simulink model "dft_8_point"  (R2016b)
settings: Solver=VariableStepDiscrete  StartTime=0.0  StopTime=12/fs  RelTol=1e-3  EnableMultiTasking=on
PreLoadFcn:
  | t = 2;
  | b = 14;
  | 
  | fs = 1;
StartFcn:
  | close all;
StopFcn:
  | % create matrices of Re and Im parts over time - inputs
  | xin_re = [xin_0_re xin_1_re xin_2_re xin_3_re xin_4_re xin_5_re xin_6_re xin_7_re];
  | xin_im = [xin_0_im xin_0_im xin_0_im xin_0_im xin_0_im xin_0_im xin_0_im xin_0_im];
  | 
  | % create matrices of Re and Im parts over time - outputs
  | X_re = [X0_re X1_re X2_re X3_re X4_re X5_re X6_re X7_re];
  | X_im = [X0_im X1_im X2_im X3_im X4_im X5_im X6_im X7_im];
  | 
  | % create vectors of Magnitudes and Angles over time
  | X_mag = [X0_mag X1_mag X2_mag X3_mag X4_mag X5_mag X6_mag X7_mag];
  | X_ang = [X0_ang X1_ang X2_ang X3_ang X4_ang X5_ang X6_ang X7_ang];
  | 
  | 
  | figure(1)
  | hold off
  | plot([0:1:7],xin_re(end,:),'r-o','MarkerFaceColor','r');
  | hold on
  | plot([0:1:7],xin_im(end,:),'b-o','MarkerFaceColor','b');
  | xlabel('Samples');
  | ylabel('Magnitude');
  | title('Input to DFT');
  | legend('Real','Imaginary','Location','EastOutside')
  | grid on;
  | 
  | set(1,'Name','Input to DFT','NumberTitle','off');
  | % setStandardFigSize(1);
  | 
  | figure(2)
  | hold off
  | plot([0:1:7],X_mag(end,:),'k-o','MarkerFaceColor','b');
  | hold on
  | xlabel('Frequency Bin');
  | ylabel('Magnitude');
  | grid on;
  | title('Magnitude DFT Plot');
  | 
  | set(2,'Name','Output of DFT','NumberTitle','off');
  | % setStandardFigSize(2);
libraries: xbsIndex_r4 x955
(part 2 of 8)

== system dft_8_point/Capture X0 Outputs ==
  In1 : Inport
  In2 : Inport  Port=2
  Complex to Magnitude-Angle : ComplexToMagnitudeAngle
  Real-Imag to Complex : RealImagToComplex
  To Workspace : ToWorkspace  VariableName=X0_im  SampleTime=-1
  To Workspace1 : ToWorkspace  VariableName=X0_re  SampleTime=-1
  To Workspace16 : ToWorkspace  VariableName=X0_mag  SampleTime=-1
  To Workspace17 : ToWorkspace  VariableName=X0_ang  SampleTime=-1
  wires:
  In1/1 -> Real-Imag to Complex/2, To Workspace/1
  In2/1 -> Real-Imag to Complex/1, To Workspace1/1
  Real-Imag to Complex/1 -> Complex to Magnitude-Angle/1
  Complex to Magnitude-Angle/2 -> To Workspace17/1
  Complex to Magnitude-Angle/1 -> To Workspace16/1

== system dft_8_point/Capture X2 Outputs ==
  In1 : Inport
  In2 : Inport  Port=2
  Complex to Magnitude-Angle2 : ComplexToMagnitudeAngle
  Real-Imag to Complex2 : RealImagToComplex
  To Workspace20 : ToWorkspace  VariableName=X2_mag  SampleTime=-1
  To Workspace21 : ToWorkspace  VariableName=X2_ang  SampleTime=-1
  To Workspace4 : ToWorkspace  VariableName=X2_im  SampleTime=-1
  To Workspace5 : ToWorkspace  VariableName=X2_re  SampleTime=-1
  wires:
  In1/1 -> Real-Imag to Complex2/2, To Workspace4/1
  In2/1 -> Real-Imag to Complex2/1, To Workspace5/1
  Real-Imag to Complex2/1 -> Complex to Magnitude-Angle2/1
  Complex to Magnitude-Angle2/2 -> To Workspace21/1
  Complex to Magnitude-Angle2/1 -> To Workspace20/1

== system dft_8_point/Capture X6 Outputs ==
  In1 : Inport
  In2 : Inport  Port=2
  Complex to Magnitude-Angle6 : ComplexToMagnitudeAngle
  Real-Imag to Complex6 : RealImagToComplex
  To Workspace12 : ToWorkspace  VariableName=X6_im  SampleTime=-1
  To Workspace13 : ToWorkspace  VariableName=X6_re  SampleTime=-1
  To Workspace28 : ToWorkspace  VariableName=X6_mag  SampleTime=-1
  To Workspace29 : ToWorkspace  VariableName=X6_ang  SampleTime=-1
  wires:
  In1/1 -> Real-Imag to Complex6/2, To Workspace12/1
  In2/1 -> Real-Imag to Complex6/1, To Workspace13/1
  Real-Imag to Complex6/1 -> Complex to Magnitude-Angle6/1
  Complex to Magnitude-Angle6/2 -> To Workspace29/1
  Complex to Magnitude-Angle6/1 -> To Workspace28/1

== system dft_8_point/Capture X1 Outputs ==
  In1 : Inport
  In2 : Inport  Port=2
  Complex to Magnitude-Angle1 : ComplexToMagnitudeAngle
  Real-Imag to Complex1 : RealImagToComplex
  To Workspace18 : ToWorkspace  VariableName=X1_mag  SampleTime=-1
  To Workspace19 : ToWorkspace  VariableName=X1_ang  SampleTime=-1
  To Workspace2 : ToWorkspace  VariableName=X1_im  SampleTime=-1
  To Workspace3 : ToWorkspace  VariableName=X1_re  SampleTime=-1
  wires:
  In1/1 -> Real-Imag to Complex1/2, To Workspace2/1
  In2/1 -> Real-Imag to Complex1/1, To Workspace3/1
  Real-Imag to Complex1/1 -> Complex to Magnitude-Angle1/1
  Complex to Magnitude-Angle1/2 -> To Workspace19/1
  Complex to Magnitude-Angle1/1 -> To Workspace18/1

== system dft_8_point/Capture X3 Outputs ==
  In1 : Inport
  In2 : Inport  Port=2
  Complex to Magnitude-Angle3 : ComplexToMagnitudeAngle
  Real-Imag to Complex3 : RealImagToComplex
  To Workspace22 : ToWorkspace  VariableName=X3_mag  SampleTime=-1
  To Workspace23 : ToWorkspace  VariableName=X3_ang  SampleTime=-1
  To Workspace6 : ToWorkspace  VariableName=X3_im  SampleTime=-1
  To Workspace7 : ToWorkspace  VariableName=X3_re  SampleTime=-1
  wires:
  In1/1 -> Real-Imag to Complex3/2, To Workspace6/1
  In2/1 -> Real-Imag to Complex3/1, To Workspace7/1
  Real-Imag to Complex3/1 -> Complex to Magnitude-Angle3/1
  Complex to Magnitude-Angle3/2 -> To Workspace23/1
  Complex to Magnitude-Angle3/1 -> To Workspace22/1

== system dft_8_point/Capture X4 Outputs ==
  In1 : Inport
  In2 : Inport  Port=2
  Complex to Magnitude-Angle4 : ComplexToMagnitudeAngle
  Real-Imag to Complex4 : RealImagToComplex
  To Workspace24 : ToWorkspace  VariableName=X4_mag  SampleTime=-1
  To Workspace25 : ToWorkspace  VariableName=X4_ang  SampleTime=-1
  To Workspace8 : ToWorkspace  VariableName=X4_im  SampleTime=-1
  To Workspace9 : ToWorkspace  VariableName=X4_re  SampleTime=-1
  wires:
  In1/1 -> Real-Imag to Complex4/2, To Workspace8/1
  In2/1 -> Real-Imag to Complex4/1, To Workspace9/1
  Real-Imag to Complex4/1 -> Complex to Magnitude-Angle4/1
  Complex to Magnitude-Angle4/2 -> To Workspace25/1
  Complex to Magnitude-Angle4/1 -> To Workspace24/1

== system dft_8_point/Capture X5 Outputs ==
  In1 : Inport
  In2 : Inport  Port=2
  Complex to Magnitude-Angle5 : ComplexToMagnitudeAngle
  Real-Imag to Complex5 : RealImagToComplex
  To Workspace10 : ToWorkspace  VariableName=X5_im  SampleTime=-1
  To Workspace11 : ToWorkspace  VariableName=X5_re  SampleTime=-1
  To Workspace26 : ToWorkspace  VariableName=X5_mag  SampleTime=-1
  To Workspace27 : ToWorkspace  VariableName=X5_ang  SampleTime=-1
  wires:
  In1/1 -> Real-Imag to Complex5/2, To Workspace10/1
  In2/1 -> Real-Imag to Complex5/1, To Workspace11/1
  Real-Imag to Complex5/1 -> Complex to Magnitude-Angle5/1
  Complex to Magnitude-Angle5/2 -> To Workspace27/1
  Complex to Magnitude-Angle5/1 -> To Workspace26/1

== system dft_8_point/Capture X7 Outputs ==
  In1 : Inport
  In2 : Inport  Port=2
  Complex to Magnitude-Angle7 : ComplexToMagnitudeAngle
  Real-Imag to Complex7 : RealImagToComplex
  To Workspace14 : ToWorkspace  VariableName=X7_im  SampleTime=-1
  To Workspace15 : ToWorkspace  VariableName=X7_re  SampleTime=-1
  To Workspace30 : ToWorkspace  VariableName=X7_mag  SampleTime=-1
  To Workspace31 : ToWorkspace  VariableName=X7_ang  SampleTime=-1
  wires:
  In1/1 -> Real-Imag to Complex7/2, To Workspace14/1
  In2/1 -> Real-Imag to Complex7/1, To Workspace15/1
  Real-Imag to Complex7/1 -> Complex to Magnitude-Angle7/1
  Complex to Magnitude-Angle7/2 -> To Workspace31/1
  Complex to Magnitude-Angle7/1 -> To Workspace30/1

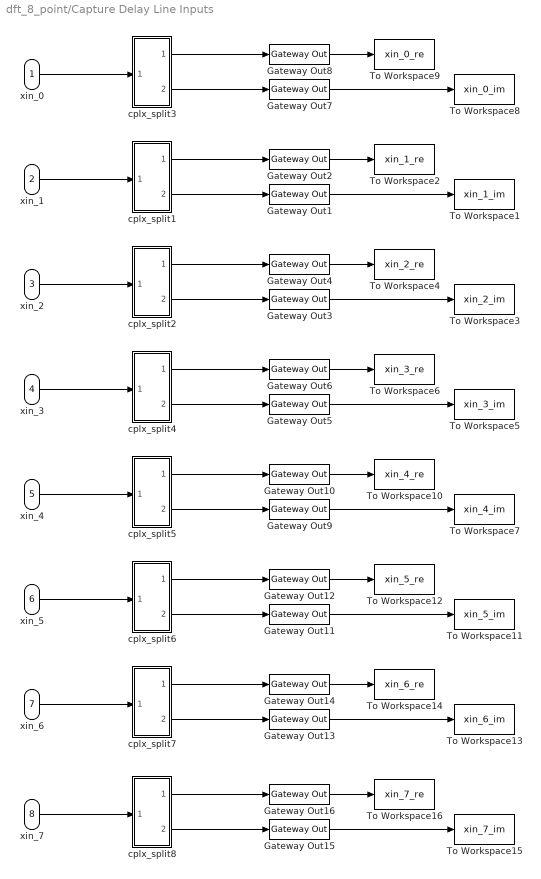
== system dft_8_point/Capture Delay Line Inputs ==
  xin_0 : Inport
  xin_1 : Inport  Port=2
  xin_2 : Inport  Port=3
  xin_3 : Inport  Port=4
  xin_4 : Inport  Port=5
  xin_5 : Inport  Port=6
  xin_6 : Inport  Port=7
  xin_7 : Inport  Port=8
  Gateway Out{1..16} (16 alike) : xbsIndex_r4/Gateway Out  inherit_from_input=off  hdl_port=off  rows=1  columns=1  UseAsDAC=off  DACChannel='1'  interface=None  automatic_assignment=on  address_offset=hex2dec('00')  intf_name=''  intf_description=''  timing_constraint=None  locs_specified=off  LOCs={}  io_standard={}  block_type=gatewayout
      settings: infoedit="Gateway out block.  Converts Xilinx fixed point inputs into ouputs of type Simulink integer, double, or fixed point.<br><br>Hardware notes:  In hardware these blocks become top level output ports or are discarded, depending on how they are configured."
  To Workspace1 : ToWorkspace  VariableName=xin_1_im  SampleTime=-1
  To Workspace10 : ToWorkspace  VariableName=xin_4_re  SampleTime=-1
  To Workspace11 : ToWorkspace  VariableName=xin_5_im  SampleTime=-1
  To Workspace12 : ToWorkspace  VariableName=xin_5_re  SampleTime=-1
  To Workspace13 : ToWorkspace  VariableName=xin_6_im  SampleTime=-1
  To Workspace14 : ToWorkspace  VariableName=xin_6_re  SampleTime=-1
  To Workspace15 : ToWorkspace  VariableName=xin_7_im  SampleTime=-1
  To Workspace16 : ToWorkspace  VariableName=xin_7_re  SampleTime=-1
  To Workspace2 : ToWorkspace  VariableName=xin_1_re  SampleTime=-1
  To Workspace3 : ToWorkspace  VariableName=xin_2_im  SampleTime=-1
  To Workspace4 : ToWorkspace  VariableName=xin_2_re  SampleTime=-1
  To Workspace5 : ToWorkspace  VariableName=xin_3_im  SampleTime=-1
  To Workspace6 : ToWorkspace  VariableName=xin_3_re  SampleTime=-1
  To Workspace7 : ToWorkspace  VariableName=xin_4_im  SampleTime=-1
  To Workspace8 : ToWorkspace  VariableName=xin_0_im  SampleTime=-1
  To Workspace9 : ToWorkspace  VariableName=xin_0_re  SampleTime=-1
  cplx_split1 : Subsystem  mask(Complex to Real / Imaginary){t=t, b=b}
      mask prompts: t "Input integer bits"; b "Input fractional bits"
      mask help:
      | This block converts the signal from a signal complex one {real,imaginary} to separate parts.
      |
      | The integer and fractional wordlengths of the real and imaginary parts are supplied so that the combined word can be separated.
  cplx_split2 : Subsystem  mask(Complex to Real / Imaginary){t=t, b=b}
      mask prompts: t "Input integer bits"; b "Input fractional bits"
      mask help:
      | This block converts the signal from a signal complex one {real,imaginary} to separate parts.
      |
      | The integer and fractional wordlengths of the real and imaginary parts are supplied so that the combined word can be separated.
  cplx_split3 : Subsystem  mask(Complex to Real / Imaginary){t=t, b=b}
      mask prompts: t "Input integer bits"; b "Input fractional bits"
      mask help:
      | This block converts the signal from a signal complex one {real,imaginary} to separate parts.
      |
      | The integer and fractional wordlengths of the real and imaginary parts are supplied so that the combined word can be separated.
  cplx_split4 : Subsystem  mask(Complex to Real / Imaginary){t=t, b=b}
      mask prompts: t "Input integer bits"; b "Input fractional bits"
      mask help:
      | This block converts the signal from a signal complex one {real,imaginary} to separate parts.
      |
      | The integer and fractional wordlengths of the real and imaginary parts are supplied so that the combined word can be separated.
  cplx_split5 : Subsystem  mask(Complex to Real / Imaginary){t=t, b=b}
      mask prompts: t "Input integer bits"; b "Input fractional bits"
      mask help:
      | This block converts the signal from a signal complex one {real,imaginary} to separate parts.
      |
      | The integer and fractional wordlengths of the real and imaginary parts are supplied so that the combined word can be separated.
  cplx_split6 : Subsystem  mask(Complex to Real / Imaginary){t=t, b=b}
      mask prompts: t "Input integer bits"; b "Input fractional bits"
      mask help:
      | This block converts the signal from a signal complex one {real,imaginary} to separate parts.
      |
      | The integer and fractional wordlengths of the real and imaginary parts are supplied so that the combined word can be separated.
  cplx_split7 : Subsystem  mask(Complex to Real / Imaginary){t=t, b=b}
      mask prompts: t "Input integer bits"; b "Input fractional bits"
      mask help:
      | This block converts the signal from a signal complex one {real,imaginary} to separate parts.
      |
      | The integer and fractional wordlengths of the real and imaginary parts are supplied so that the combined word can be separated.
  cplx_split8 : Subsystem  mask(Complex to Real / Imaginary){t=t, b=b}
      mask prompts: t "Input integer bits"; b "Input fractional bits"
      mask help:
      | This block converts the signal from a signal complex one {real,imaginary} to separate parts.
      |
      | The integer and fractional wordlengths of the real and imaginary parts are supplied so that the combined word can be separated.
  wires:
  xin_0/1 -> cplx_split3/1(cmplx)
  xin_1/1 -> cplx_split1/1(cmplx)
  xin_2/1 -> cplx_split2/1(cmplx)
  xin_3/1 -> cplx_split4/1(cmplx)
  xin_4/1 -> cplx_split5/1(cmplx)
  xin_5/1 -> cplx_split6/1(cmplx)
  xin_6/1 -> cplx_split7/1(cmplx)
  xin_7/1 -> cplx_split8/1(cmplx)
  cplx_split3/1(real) -> Gateway Out8/1
  cplx_split3/2(imag) -> Gateway Out7/1
  Gateway Out7/1 -> To Workspace8/1
  Gateway Out8/1 -> To Workspace9/1
  cplx_split1/1(real) -> Gateway Out2/1
  cplx_split1/2(imag) -> Gateway Out1/1
  Gateway Out1/1 -> To Workspace1/1
  Gateway Out2/1 -> To Workspace2/1
  cplx_split2/1(real) -> Gateway Out4/1
  cplx_split2/2(imag) -> Gateway Out3/1
  Gateway Out3/1 -> To Workspace3/1
  Gateway Out4/1 -> To Workspace4/1
  cplx_split4/1(real) -> Gateway Out6/1
  cplx_split4/2(imag) -> Gateway Out5/1
  Gateway Out5/1 -> To Workspace5/1
  Gateway Out6/1 -> To Workspace6/1
  cplx_split5/1(real) -> Gateway Out10/1
  cplx_split5/2(imag) -> Gateway Out9/1
  Gateway Out9/1 -> To Workspace7/1
  Gateway Out10/1 -> To Workspace10/1
  cplx_split6/1(real) -> Gateway Out12/1
  cplx_split6/2(imag) -> Gateway Out11/1
  Gateway Out11/1 -> To Workspace11/1
  Gateway Out12/1 -> To Workspace12/1
  cplx_split7/1(real) -> Gateway Out14/1
  cplx_split7/2(imag) -> Gateway Out13/1
  Gateway Out13/1 -> To Workspace13/1
  Gateway Out14/1 -> To Workspace14/1
  cplx_split8/1(real) -> Gateway Out16/1
  cplx_split8/2(imag) -> Gateway Out15/1
  Gateway Out15/1 -> To Workspace15/1
  Gateway Out16/1 -> To Workspace16/1

== system dft_8_point/See: File -> Model Properties -> Callbacks -> PreLoadFcn  ==

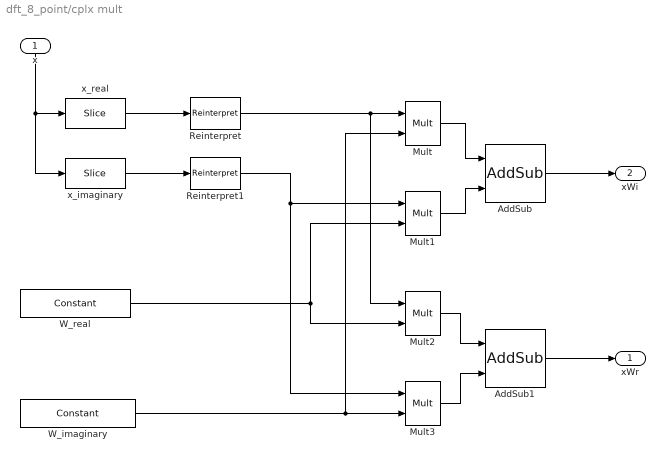
== system dft_8_point/cplx mult ==
  x : Inport
  AddSub : xbsIndex_r4/AddSub  mode=Addition  use_carryin=off  use_carryout=off  en=off  latency=0  precision=User Defined  arith_type="Signed  (2's comp)"  n_bits=t+b+1  bin_pt=b  quantization=Truncate  overflow=Wrap  use_behavioral_HDL=off  hw_selection=Fabric  pipelined=off  dbl_ovrd=off  block_type=addsub
  AddSub1 : xbsIndex_r4/AddSub  mode=Subtraction  use_carryin=off  use_carryout=off  en=off  latency=0  precision=User Defined  arith_type="Signed  (2's comp)"  n_bits=t+b+1  bin_pt=b  quantization=Truncate  overflow=Wrap  use_behavioral_HDL=off  hw_selection=Fabric  pipelined=off  dbl_ovrd=off  block_type=addsub
  Mult{,1..3} (4 alike) : xbsIndex_r4/Mult  precision=User Defined  arith_type="Signed  (2's comp)"  n_bits=t+b  bin_pt=b  quantization=Truncate  overflow=Wrap  en=off  latency=0  use_behavioral_HDL=off  opt=Speed  use_embedded=on  optimum_pipeline=off  pipeline=on  dbl_ovrd=off  use_rpm=on  placement_style=Triangular  block_type=mult
  Reinterpret : xbsIndex_r4/Reinterpret  force_arith_type=on  arith_type="Signed  (2's comp)"  force_bin_pt=on  bin_pt=b  block_type=reinterpret
      settings: infoedit="Changes signal type without altering the binary representation.   You can changed the signal between signed and unsigned, and relocate the binary point.<br><br>Hardware notes: In hardware this block costs nothing.<br><br>Example:  Suppose the input is 6 bits wide, signed, with 2 fractional bits, and the output is forced to unsigned with 0 fractional bits.  Then an input of -2.0 (1110.00 in binary 2's complement) becomes an output of 56 (111000 in binary)."
  Reinterpret1 : xbsIndex_r4/Reinterpret  force_arith_type=on  arith_type="Signed  (2's comp)"  force_bin_pt=on  bin_pt=b  block_type=reinterpret
      settings: infoedit="Changes signal type without altering the binary representation.   You can changed the signal between signed and unsigned, and relocate the binary point.<br><br>Hardware notes: In hardware this block costs nothing.<br><br>Example:  Suppose the input is 6 bits wide, signed, with 2 fractional bits, and the output is forced to unsigned with 0 fractional bits.  Then an input of -2.0 (1110.00 in binary 2's complement) becomes an output of 56 (111000 in binary)."
  W_imaginary : xbsIndex_r4/Constant  const=imag(Wnk)  gui_display_data_type=Fixed-point  arith_type=Signed (2's comp)  n_bits=t+b  bin_pt=b  preci_type=Single  exp_width=8  frac_width=24  explicit_period=off  period=1  equ=P=C  opselect=C  inp2=PCIN>>17  opr=+  inp1=P  carry=CIN  dbl_ovrd=off  block_type=constant
  W_real : xbsIndex_r4/Constant  const=real(Wnk)  gui_display_data_type=Fixed-point  arith_type=Signed (2's comp)  n_bits=t+b  bin_pt=b  preci_type=Single  exp_width=8  frac_width=24  explicit_period=off  period=1  equ=P=C  opselect=C  inp2=PCIN>>17  opr=+  inp1=P  carry=CIN  dbl_ovrd=off  block_type=constant
  x_imaginary : xbsIndex_r4/Slice  nbits=t+b  boolean_output=off  mode=Lower Bit Location + Width  bit1=0  base1=MSB of Input  bit0=0  base0=LSB of Input  dbl_ovrd=off  block_type=slice
  x_real : xbsIndex_r4/Slice  nbits=t+b  boolean_output=off  mode=Upper Bit Location + Width  bit1=0  base1=MSB of Input  bit0=0  base0=LSB of Input  dbl_ovrd=off  block_type=slice
  xWr : Outport
  xWi : Outport  Port=2
  wires:
  x_real/1 -> Reinterpret/1
  x_imaginary/1 -> Reinterpret1/1
  W_real/1 -> Mult1/2, Mult2/2
  x/1 -> x_real/1, x_imaginary/1
  Reinterpret/1 -> Mult/1, Mult2/1
  Reinterpret1/1 -> Mult1/1, Mult3/1
  W_imaginary/1 -> Mult/2, Mult3/2
  AddSub/1 -> xWi/1
  AddSub1/1 -> xWr/1
  Mult/1 -> AddSub/1
  Mult1/1 -> AddSub/2
  Mult3/1 -> AddSub1/2
  Mult2/1 -> AddSub1/1

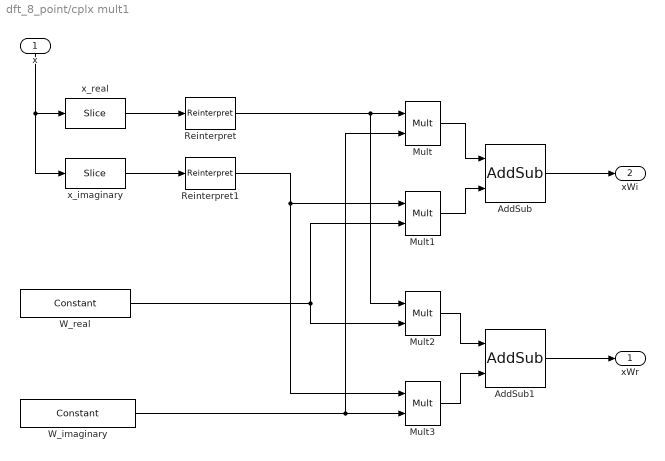
== system dft_8_point/cplx mult1 ==
  x : Inport
  AddSub : xbsIndex_r4/AddSub  mode=Addition  use_carryin=off  use_carryout=off  en=off  latency=0  precision=User Defined  arith_type="Signed  (2's comp)"  n_bits=t+b+1  bin_pt=b  quantization=Truncate  overflow=Wrap  use_behavioral_HDL=off  hw_selection=Fabric  pipelined=off  dbl_ovrd=off  block_type=addsub
  AddSub1 : xbsIndex_r4/AddSub  mode=Subtraction  use_carryin=off  use_carryout=off  en=off  latency=0  precision=User Defined  arith_type="Signed  (2's comp)"  n_bits=t+b+1  bin_pt=b  quantization=Truncate  overflow=Wrap  use_behavioral_HDL=off  hw_selection=Fabric  pipelined=off  dbl_ovrd=off  block_type=addsub
  Mult{,1..3} (4 alike) : xbsIndex_r4/Mult  precision=User Defined  arith_type="Signed  (2's comp)"  n_bits=t+b  bin_pt=b  quantization=Truncate  overflow=Wrap  en=off  latency=0  use_behavioral_HDL=off  opt=Speed  use_embedded=on  optimum_pipeline=off  pipeline=on  dbl_ovrd=off  use_rpm=on  placement_style=Triangular  block_type=mult
  Reinterpret : xbsIndex_r4/Reinterpret  force_arith_type=on  arith_type="Signed  (2's comp)"  force_bin_pt=on  bin_pt=b  block_type=reinterpret
      settings: infoedit="Changes signal type without altering the binary representation.   You can changed the signal between signed and unsigned, and relocate the binary point.<br><br>Hardware notes: In hardware this block costs nothing.<br><br>Example:  Suppose the input is 6 bits wide, signed, with 2 fractional bits, and the output is forced to unsigned with 0 fractional bits.  Then an input of -2.0 (1110.00 in binary 2's complement) becomes an output of 56 (111000 in binary)."
  Reinterpret1 : xbsIndex_r4/Reinterpret  force_arith_type=on  arith_type="Signed  (2's comp)"  force_bin_pt=on  bin_pt=b  block_type=reinterpret
      settings: infoedit="Changes signal type without altering the binary representation.   You can changed the signal between signed and unsigned, and relocate the binary point.<br><br>Hardware notes: In hardware this block costs nothing.<br><br>Example:  Suppose the input is 6 bits wide, signed, with 2 fractional bits, and the output is forced to unsigned with 0 fractional bits.  Then an input of -2.0 (1110.00 in binary 2's complement) becomes an output of 56 (111000 in binary)."
  W_imaginary : xbsIndex_r4/Constant  const=imag(Wnk)  gui_display_data_type=Fixed-point  arith_type=Signed (2's comp)  n_bits=t+b  bin_pt=b  preci_type=Single  exp_width=8  frac_width=24  explicit_period=off  period=1  equ=P=C  opselect=C  inp2=PCIN>>17  opr=+  inp1=P  carry=CIN  dbl_ovrd=off  block_type=constant
  W_real : xbsIndex_r4/Constant  const=real(Wnk)  gui_display_data_type=Fixed-point  arith_type=Signed (2's comp)  n_bits=t+b  bin_pt=b  preci_type=Single  exp_width=8  frac_width=24  explicit_period=off  period=1  equ=P=C  opselect=C  inp2=PCIN>>17  opr=+  inp1=P  carry=CIN  dbl_ovrd=off  block_type=constant
  x_imaginary : xbsIndex_r4/Slice  nbits=t+b  boolean_output=off  mode=Lower Bit Location + Width  bit1=0  base1=MSB of Input  bit0=0  base0=LSB of Input  dbl_ovrd=off  block_type=slice
  x_real : xbsIndex_r4/Slice  nbits=t+b  boolean_output=off  mode=Upper Bit Location + Width  bit1=0  base1=MSB of Input  bit0=0  base0=LSB of Input  dbl_ovrd=off  block_type=slice
  xWr : Outport
  xWi : Outport  Port=2
  wires:
  x_real/1 -> Reinterpret/1
  x_imaginary/1 -> Reinterpret1/1
  W_real/1 -> Mult1/2, Mult2/2
  x/1 -> x_real/1, x_imaginary/1
  Reinterpret/1 -> Mult/1, Mult2/1
  Reinterpret1/1 -> Mult1/1, Mult3/1
  W_imaginary/1 -> Mult/2, Mult3/2
  AddSub/1 -> xWi/1
  AddSub1/1 -> xWr/1
  Mult/1 -> AddSub/1
  Mult1/1 -> AddSub/2
  Mult3/1 -> AddSub1/2
  Mult2/1 -> AddSub1/1

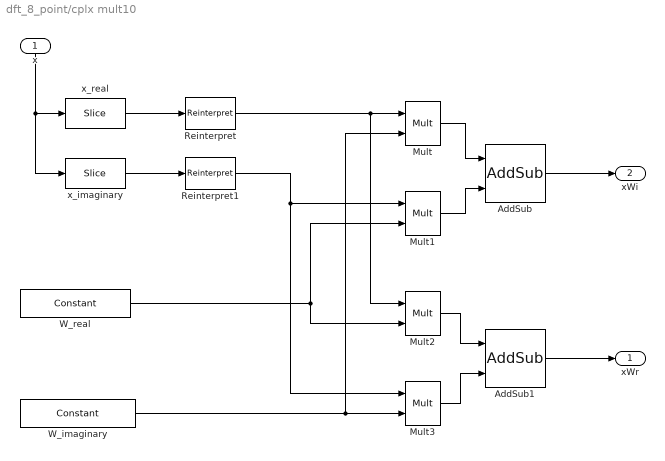
== system dft_8_point/cplx mult10 ==
  x : Inport
  AddSub : xbsIndex_r4/AddSub  mode=Addition  use_carryin=off  use_carryout=off  en=off  latency=0  precision=User Defined  arith_type="Signed  (2's comp)"  n_bits=t+b+1  bin_pt=b  quantization=Truncate  overflow=Wrap  use_behavioral_HDL=off  hw_selection=Fabric  pipelined=off  dbl_ovrd=off  block_type=addsub
  AddSub1 : xbsIndex_r4/AddSub  mode=Subtraction  use_carryin=off  use_carryout=off  en=off  latency=0  precision=User Defined  arith_type="Signed  (2's comp)"  n_bits=t+b+1  bin_pt=b  quantization=Truncate  overflow=Wrap  use_behavioral_HDL=off  hw_selection=Fabric  pipelined=off  dbl_ovrd=off  block_type=addsub
  Mult{,1..3} (4 alike) : xbsIndex_r4/Mult  precision=User Defined  arith_type="Signed  (2's comp)"  n_bits=t+b  bin_pt=b  quantization=Truncate  overflow=Wrap  en=off  latency=0  use_behavioral_HDL=off  opt=Speed  use_embedded=on  optimum_pipeline=off  pipeline=on  dbl_ovrd=off  use_rpm=on  placement_style=Triangular  block_type=mult
  Reinterpret : xbsIndex_r4/Reinterpret  force_arith_type=on  arith_type="Signed  (2's comp)"  force_bin_pt=on  bin_pt=b  block_type=reinterpret
      settings: infoedit="Changes signal type without altering the binary representation.   You can changed the signal between signed and unsigned, and relocate the binary point.<br><br>Hardware notes: In hardware this block costs nothing.<br><br>Example:  Suppose the input is 6 bits wide, signed, with 2 fractional bits, and the output is forced to unsigned with 0 fractional bits.  Then an input of -2.0 (1110.00 in binary 2's complement) becomes an output of 56 (111000 in binary)."
  Reinterpret1 : xbsIndex_r4/Reinterpret  force_arith_type=on  arith_type="Signed  (2's comp)"  force_bin_pt=on  bin_pt=b  block_type=reinterpret
      settings: infoedit="Changes signal type without altering the binary representation.   You can changed the signal between signed and unsigned, and relocate the binary point.<br><br>Hardware notes: In hardware this block costs nothing.<br><br>Example:  Suppose the input is 6 bits wide, signed, with 2 fractional bits, and the output is forced to unsigned with 0 fractional bits.  Then an input of -2.0 (1110.00 in binary 2's complement) becomes an output of 56 (111000 in binary)."
  W_imaginary : xbsIndex_r4/Constant  const=imag(Wnk)  gui_display_data_type=Fixed-point  arith_type=Signed (2's comp)  n_bits=t+b  bin_pt=b  preci_type=Single  exp_width=8  frac_width=24  explicit_period=off  period=1  equ=P=C  opselect=C  inp2=PCIN>>17  opr=+  inp1=P  carry=CIN  dbl_ovrd=off  block_type=constant
  W_real : xbsIndex_r4/Constant  const=real(Wnk)  gui_display_data_type=Fixed-point  arith_type=Signed (2's comp)  n_bits=t+b  bin_pt=b  preci_type=Single  exp_width=8  frac_width=24  explicit_period=off  period=1  equ=P=C  opselect=C  inp2=PCIN>>17  opr=+  inp1=P  carry=CIN  dbl_ovrd=off  block_type=constant
  x_imaginary : xbsIndex_r4/Slice  nbits=t+b  boolean_output=off  mode=Lower Bit Location + Width  bit1=0  base1=MSB of Input  bit0=0  base0=LSB of Input  dbl_ovrd=off  block_type=slice
  x_real : xbsIndex_r4/Slice  nbits=t+b  boolean_output=off  mode=Upper Bit Location + Width  bit1=0  base1=MSB of Input  bit0=0  base0=LSB of Input  dbl_ovrd=off  block_type=slice
  xWr : Outport
  xWi : Outport  Port=2
  wires:
  x_real/1 -> Reinterpret/1
  x_imaginary/1 -> Reinterpret1/1
  W_real/1 -> Mult1/2, Mult2/2
  x/1 -> x_real/1, x_imaginary/1
  Reinterpret/1 -> Mult/1, Mult2/1
  Reinterpret1/1 -> Mult1/1, Mult3/1
  W_imaginary/1 -> Mult/2, Mult3/2
  AddSub/1 -> xWi/1
  AddSub1/1 -> xWr/1
  Mult/1 -> AddSub/1
  Mult1/1 -> AddSub/2
  Mult3/1 -> AddSub1/2
  Mult2/1 -> AddSub1/1

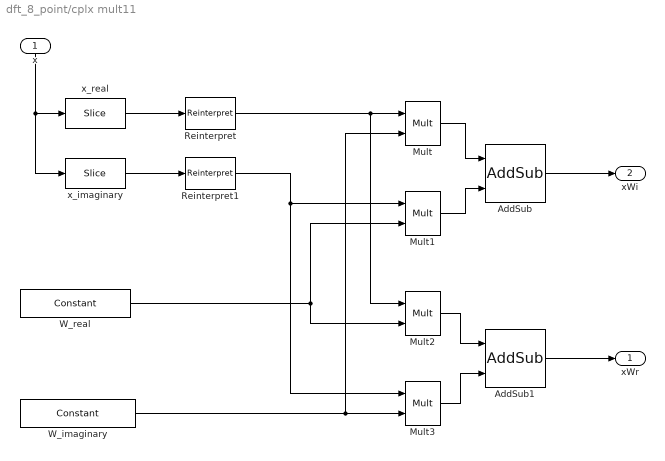
== system dft_8_point/cplx mult11 ==
  x : Inport
  AddSub : xbsIndex_r4/AddSub  mode=Addition  use_carryin=off  use_carryout=off  en=off  latency=0  precision=User Defined  arith_type="Signed  (2's comp)"  n_bits=t+b+1  bin_pt=b  quantization=Truncate  overflow=Wrap  use_behavioral_HDL=off  hw_selection=Fabric  pipelined=off  dbl_ovrd=off  block_type=addsub
  AddSub1 : xbsIndex_r4/AddSub  mode=Subtraction  use_carryin=off  use_carryout=off  en=off  latency=0  precision=User Defined  arith_type="Signed  (2's comp)"  n_bits=t+b+1  bin_pt=b  quantization=Truncate  overflow=Wrap  use_behavioral_HDL=off  hw_selection=Fabric  pipelined=off  dbl_ovrd=off  block_type=addsub
  Mult{,1..3} (4 alike) : xbsIndex_r4/Mult  precision=User Defined  arith_type="Signed  (2's comp)"  n_bits=t+b  bin_pt=b  quantization=Truncate  overflow=Wrap  en=off  latency=0  use_behavioral_HDL=off  opt=Speed  use_embedded=on  optimum_pipeline=off  pipeline=on  dbl_ovrd=off  use_rpm=on  placement_style=Triangular  block_type=mult
  Reinterpret : xbsIndex_r4/Reinterpret  force_arith_type=on  arith_type="Signed  (2's comp)"  force_bin_pt=on  bin_pt=b  block_type=reinterpret
      settings: infoedit="Changes signal type without altering the binary representation.   You can changed the signal between signed and unsigned, and relocate the binary point.<br><br>Hardware notes: In hardware this block costs nothing.<br><br>Example:  Suppose the input is 6 bits wide, signed, with 2 fractional bits, and the output is forced to unsigned with 0 fractional bits.  Then an input of -2.0 (1110.00 in binary 2's complement) becomes an output of 56 (111000 in binary)."
  Reinterpret1 : xbsIndex_r4/Reinterpret  force_arith_type=on  arith_type="Signed  (2's comp)"  force_bin_pt=on  bin_pt=b  block_type=reinterpret
      settings: infoedit="Changes signal type without altering the binary representation.   You can changed the signal between signed and unsigned, and relocate the binary point.<br><br>Hardware notes: In hardware this block costs nothing.<br><br>Example:  Suppose the input is 6 bits wide, signed, with 2 fractional bits, and the output is forced to unsigned with 0 fractional bits.  Then an input of -2.0 (1110.00 in binary 2's complement) becomes an output of 56 (111000 in binary)."
  W_imaginary : xbsIndex_r4/Constant  const=imag(Wnk)  gui_display_data_type=Fixed-point  arith_type=Signed (2's comp)  n_bits=t+b  bin_pt=b  preci_type=Single  exp_width=8  frac_width=24  explicit_period=off  period=1  equ=P=C  opselect=C  inp2=PCIN>>17  opr=+  inp1=P  carry=CIN  dbl_ovrd=off  block_type=constant
  W_real : xbsIndex_r4/Constant  const=real(Wnk)  gui_display_data_type=Fixed-point  arith_type=Signed (2's comp)  n_bits=t+b  bin_pt=b  preci_type=Single  exp_width=8  frac_width=24  explicit_period=off  period=1  equ=P=C  opselect=C  inp2=PCIN>>17  opr=+  inp1=P  carry=CIN  dbl_ovrd=off  block_type=constant
  x_imaginary : xbsIndex_r4/Slice  nbits=t+b  boolean_output=off  mode=Lower Bit Location + Width  bit1=0  base1=MSB of Input  bit0=0  base0=LSB of Input  dbl_ovrd=off  block_type=slice
  x_real : xbsIndex_r4/Slice  nbits=t+b  boolean_output=off  mode=Upper Bit Location + Width  bit1=0  base1=MSB of Input  bit0=0  base0=LSB of Input  dbl_ovrd=off  block_type=slice
  xWr : Outport
  xWi : Outport  Port=2
  wires:
  x_real/1 -> Reinterpret/1
  x_imaginary/1 -> Reinterpret1/1
  W_real/1 -> Mult1/2, Mult2/2
  x/1 -> x_real/1, x_imaginary/1
  Reinterpret/1 -> Mult/1, Mult2/1
  Reinterpret1/1 -> Mult1/1, Mult3/1
  W_imaginary/1 -> Mult/2, Mult3/2
  AddSub/1 -> xWi/1
  AddSub1/1 -> xWr/1
  Mult/1 -> AddSub/1
  Mult1/1 -> AddSub/2
  Mult3/1 -> AddSub1/2
  Mult2/1 -> AddSub1/1

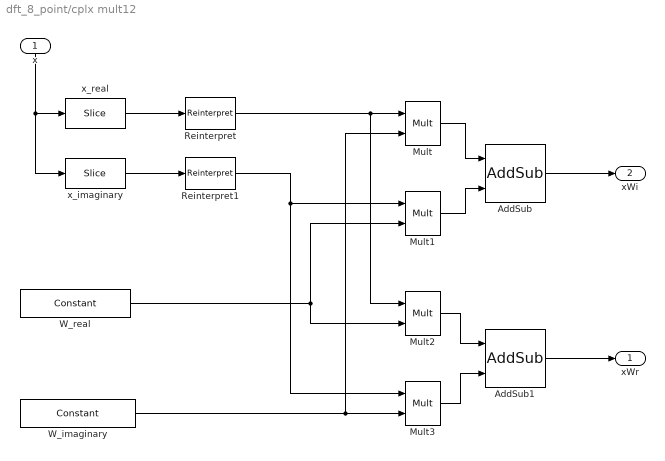
== system dft_8_point/cplx mult12 ==
  x : Inport
  AddSub : xbsIndex_r4/AddSub  mode=Addition  use_carryin=off  use_carryout=off  en=off  latency=0  precision=User Defined  arith_type="Signed  (2's comp)"  n_bits=t+b+1  bin_pt=b  quantization=Truncate  overflow=Wrap  use_behavioral_HDL=off  hw_selection=Fabric  pipelined=off  dbl_ovrd=off  block_type=addsub
  AddSub1 : xbsIndex_r4/AddSub  mode=Subtraction  use_carryin=off  use_carryout=off  en=off  latency=0  precision=User Defined  arith_type="Signed  (2's comp)"  n_bits=t+b+1  bin_pt=b  quantization=Truncate  overflow=Wrap  use_behavioral_HDL=off  hw_selection=Fabric  pipelined=off  dbl_ovrd=off  block_type=addsub
  Mult{,1..3} (4 alike) : xbsIndex_r4/Mult  precision=User Defined  arith_type="Signed  (2's comp)"  n_bits=t+b  bin_pt=b  quantization=Truncate  overflow=Wrap  en=off  latency=0  use_behavioral_HDL=off  opt=Speed  use_embedded=on  optimum_pipeline=off  pipeline=on  dbl_ovrd=off  use_rpm=on  placement_style=Triangular  block_type=mult
  Reinterpret : xbsIndex_r4/Reinterpret  force_arith_type=on  arith_type="Signed  (2's comp)"  force_bin_pt=on  bin_pt=b  block_type=reinterpret
      settings: infoedit="Changes signal type without altering the binary representation.   You can changed the signal between signed and unsigned, and relocate the binary point.<br><br>Hardware notes: In hardware this block costs nothing.<br><br>Example:  Suppose the input is 6 bits wide, signed, with 2 fractional bits, and the output is forced to unsigned with 0 fractional bits.  Then an input of -2.0 (1110.00 in binary 2's complement) becomes an output of 56 (111000 in binary)."
  Reinterpret1 : xbsIndex_r4/Reinterpret  force_arith_type=on  arith_type="Signed  (2's comp)"  force_bin_pt=on  bin_pt=b  block_type=reinterpret
      settings: infoedit="Changes signal type without altering the binary representation.   You can changed the signal between signed and unsigned, and relocate the binary point.<br><br>Hardware notes: In hardware this block costs nothing.<br><br>Example:  Suppose the input is 6 bits wide, signed, with 2 fractional bits, and the output is forced to unsigned with 0 fractional bits.  Then an input of -2.0 (1110.00 in binary 2's complement) becomes an output of 56 (111000 in binary)."
  W_imaginary : xbsIndex_r4/Constant  const=imag(Wnk)  gui_display_data_type=Fixed-point  arith_type=Signed (2's comp)  n_bits=t+b  bin_pt=b  preci_type=Single  exp_width=8  frac_width=24  explicit_period=off  period=1  equ=P=C  opselect=C  inp2=PCIN>>17  opr=+  inp1=P  carry=CIN  dbl_ovrd=off  block_type=constant
  W_real : xbsIndex_r4/Constant  const=real(Wnk)  gui_display_data_type=Fixed-point  arith_type=Signed (2's comp)  n_bits=t+b  bin_pt=b  preci_type=Single  exp_width=8  frac_width=24  explicit_period=off  period=1  equ=P=C  opselect=C  inp2=PCIN>>17  opr=+  inp1=P  carry=CIN  dbl_ovrd=off  block_type=constant
  x_imaginary : xbsIndex_r4/Slice  nbits=t+b  boolean_output=off  mode=Lower Bit Location + Width  bit1=0  base1=MSB of Input  bit0=0  base0=LSB of Input  dbl_ovrd=off  block_type=slice
  x_real : xbsIndex_r4/Slice  nbits=t+b  boolean_output=off  mode=Upper Bit Location + Width  bit1=0  base1=MSB of Input  bit0=0  base0=LSB of Input  dbl_ovrd=off  block_type=slice
  xWr : Outport
  xWi : Outport  Port=2
  wires:
  x_real/1 -> Reinterpret/1
  x_imaginary/1 -> Reinterpret1/1
  W_real/1 -> Mult1/2, Mult2/2
  x/1 -> x_real/1, x_imaginary/1
  Reinterpret/1 -> Mult/1, Mult2/1
  Reinterpret1/1 -> Mult1/1, Mult3/1
  W_imaginary/1 -> Mult/2, Mult3/2
  AddSub/1 -> xWi/1
  AddSub1/1 -> xWr/1
  Mult/1 -> AddSub/1
  Mult1/1 -> AddSub/2
  Mult3/1 -> AddSub1/2
  Mult2/1 -> AddSub1/1

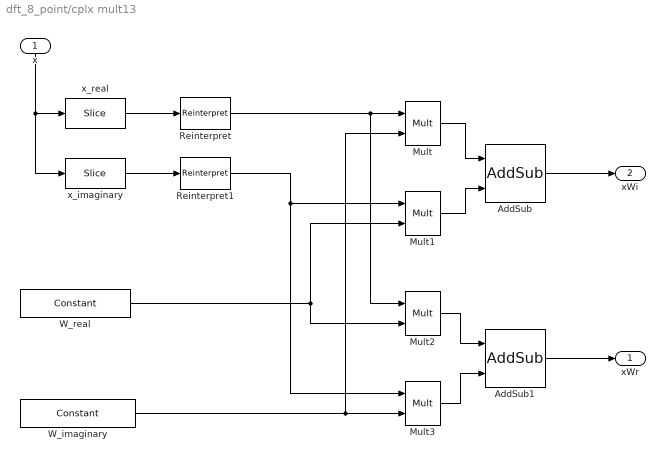
== system dft_8_point/cplx mult13 ==
  x : Inport
  AddSub : xbsIndex_r4/AddSub  mode=Addition  use_carryin=off  use_carryout=off  en=off  latency=0  precision=User Defined  arith_type="Signed  (2's comp)"  n_bits=t+b+1  bin_pt=b  quantization=Truncate  overflow=Wrap  use_behavioral_HDL=off  hw_selection=Fabric  pipelined=off  dbl_ovrd=off  block_type=addsub
  AddSub1 : xbsIndex_r4/AddSub  mode=Subtraction  use_carryin=off  use_carryout=off  en=off  latency=0  precision=User Defined  arith_type="Signed  (2's comp)"  n_bits=t+b+1  bin_pt=b  quantization=Truncate  overflow=Wrap  use_behavioral_HDL=off  hw_selection=Fabric  pipelined=off  dbl_ovrd=off  block_type=addsub
  Mult{,1..3} (4 alike) : xbsIndex_r4/Mult  precision=User Defined  arith_type="Signed  (2's comp)"  n_bits=t+b  bin_pt=b  quantization=Truncate  overflow=Wrap  en=off  latency=0  use_behavioral_HDL=off  opt=Speed  use_embedded=on  optimum_pipeline=off  pipeline=on  dbl_ovrd=off  use_rpm=on  placement_style=Triangular  block_type=mult
  Reinterpret : xbsIndex_r4/Reinterpret  force_arith_type=on  arith_type="Signed  (2's comp)"  force_bin_pt=on  bin_pt=b  block_type=reinterpret
      settings: infoedit="Changes signal type without altering the binary representation.   You can changed the signal between signed and unsigned, and relocate the binary point.<br><br>Hardware notes: In hardware this block costs nothing.<br><br>Example:  Suppose the input is 6 bits wide, signed, with 2 fractional bits, and the output is forced to unsigned with 0 fractional bits.  Then an input of -2.0 (1110.00 in binary 2's complement) becomes an output of 56 (111000 in binary)."
  Reinterpret1 : xbsIndex_r4/Reinterpret  force_arith_type=on  arith_type="Signed  (2's comp)"  force_bin_pt=on  bin_pt=b  block_type=reinterpret
      settings: infoedit="Changes signal type without altering the binary representation.   You can changed the signal between signed and unsigned, and relocate the binary point.<br><br>Hardware notes: In hardware this block costs nothing.<br><br>Example:  Suppose the input is 6 bits wide, signed, with 2 fractional bits, and the output is forced to unsigned with 0 fractional bits.  Then an input of -2.0 (1110.00 in binary 2's complement) becomes an output of 56 (111000 in binary)."
  W_imaginary : xbsIndex_r4/Constant  const=imag(Wnk)  gui_display_data_type=Fixed-point  arith_type=Signed (2's comp)  n_bits=t+b  bin_pt=b  preci_type=Single  exp_width=8  frac_width=24  explicit_period=off  period=1  equ=P=C  opselect=C  inp2=PCIN>>17  opr=+  inp1=P  carry=CIN  dbl_ovrd=off  block_type=constant
  W_real : xbsIndex_r4/Constant  const=real(Wnk)  gui_display_data_type=Fixed-point  arith_type=Signed (2's comp)  n_bits=t+b  bin_pt=b  preci_type=Single  exp_width=8  frac_width=24  explicit_period=off  period=1  equ=P=C  opselect=C  inp2=PCIN>>17  opr=+  inp1=P  carry=CIN  dbl_ovrd=off  block_type=constant
  x_imaginary : xbsIndex_r4/Slice  nbits=t+b  boolean_output=off  mode=Lower Bit Location + Width  bit1=0  base1=MSB of Input  bit0=0  base0=LSB of Input  dbl_ovrd=off  block_type=slice
  x_real : xbsIndex_r4/Slice  nbits=t+b  boolean_output=off  mode=Upper Bit Location + Width  bit1=0  base1=MSB of Input  bit0=0  base0=LSB of Input  dbl_ovrd=off  block_type=slice
  xWr : Outport
  xWi : Outport  Port=2
  wires:
  x_real/1 -> Reinterpret/1
  x_imaginary/1 -> Reinterpret1/1
  W_real/1 -> Mult1/2, Mult2/2
  x/1 -> x_real/1, x_imaginary/1
  Reinterpret/1 -> Mult/1, Mult2/1
  Reinterpret1/1 -> Mult1/1, Mult3/1
  W_imaginary/1 -> Mult/2, Mult3/2
  AddSub/1 -> xWi/1
  AddSub1/1 -> xWr/1
  Mult/1 -> AddSub/1
  Mult1/1 -> AddSub/2
  Mult3/1 -> AddSub1/2
  Mult2/1 -> AddSub1/1

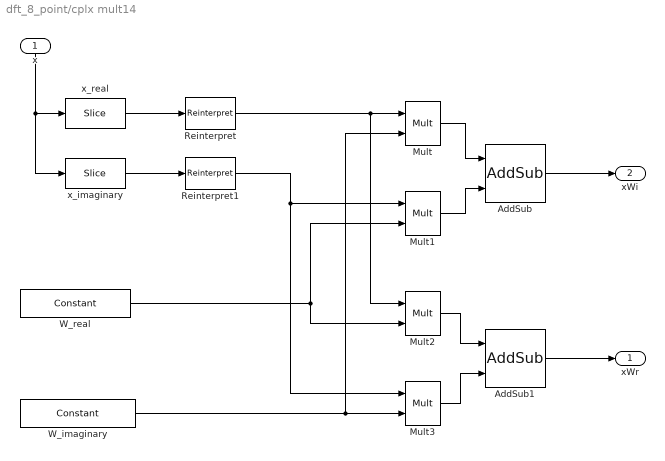
== system dft_8_point/cplx mult14 ==
  x : Inport
  AddSub : xbsIndex_r4/AddSub  mode=Addition  use_carryin=off  use_carryout=off  en=off  latency=0  precision=User Defined  arith_type="Signed  (2's comp)"  n_bits=t+b+1  bin_pt=b  quantization=Truncate  overflow=Wrap  use_behavioral_HDL=off  hw_selection=Fabric  pipelined=off  dbl_ovrd=off  block_type=addsub
  AddSub1 : xbsIndex_r4/AddSub  mode=Subtraction  use_carryin=off  use_carryout=off  en=off  latency=0  precision=User Defined  arith_type="Signed  (2's comp)"  n_bits=t+b+1  bin_pt=b  quantization=Truncate  overflow=Wrap  use_behavioral_HDL=off  hw_selection=Fabric  pipelined=off  dbl_ovrd=off  block_type=addsub
  Mult{,1..3} (4 alike) : xbsIndex_r4/Mult  precision=User Defined  arith_type="Signed  (2's comp)"  n_bits=t+b  bin_pt=b  quantization=Truncate  overflow=Wrap  en=off  latency=0  use_behavioral_HDL=off  opt=Speed  use_embedded=on  optimum_pipeline=off  pipeline=on  dbl_ovrd=off  use_rpm=on  placement_style=Triangular  block_type=mult
  Reinterpret : xbsIndex_r4/Reinterpret  force_arith_type=on  arith_type="Signed  (2's comp)"  force_bin_pt=on  bin_pt=b  block_type=reinterpret
      settings: infoedit="Changes signal type without altering the binary representation.   You can changed the signal between signed and unsigned, and relocate the binary point.<br><br>Hardware notes: In hardware this block costs nothing.<br><br>Example:  Suppose the input is 6 bits wide, signed, with 2 fractional bits, and the output is forced to unsigned with 0 fractional bits.  Then an input of -2.0 (1110.00 in binary 2's complement) becomes an output of 56 (111000 in binary)."
  Reinterpret1 : xbsIndex_r4/Reinterpret  force_arith_type=on  arith_type="Signed  (2's comp)"  force_bin_pt=on  bin_pt=b  block_type=reinterpret
      settings: infoedit="Changes signal type without altering the binary representation.   You can changed the signal between signed and unsigned, and relocate the binary point.<br><br>Hardware notes: In hardware this block costs nothing.<br><br>Example:  Suppose the input is 6 bits wide, signed, with 2 fractional bits, and the output is forced to unsigned with 0 fractional bits.  Then an input of -2.0 (1110.00 in binary 2's complement) becomes an output of 56 (111000 in binary)."
  W_imaginary : xbsIndex_r4/Constant  const=imag(Wnk)  gui_display_data_type=Fixed-point  arith_type=Signed (2's comp)  n_bits=t+b  bin_pt=b  preci_type=Single  exp_width=8  frac_width=24  explicit_period=off  period=1  equ=P=C  opselect=C  inp2=PCIN>>17  opr=+  inp1=P  carry=CIN  dbl_ovrd=off  block_type=constant
  W_real : xbsIndex_r4/Constant  const=real(Wnk)  gui_display_data_type=Fixed-point  arith_type=Signed (2's comp)  n_bits=t+b  bin_pt=b  preci_type=Single  exp_width=8  frac_width=24  explicit_period=off  period=1  equ=P=C  opselect=C  inp2=PCIN>>17  opr=+  inp1=P  carry=CIN  dbl_ovrd=off  block_type=constant
  x_imaginary : xbsIndex_r4/Slice  nbits=t+b  boolean_output=off  mode=Lower Bit Location + Width  bit1=0  base1=MSB of Input  bit0=0  base0=LSB of Input  dbl_ovrd=off  block_type=slice
  x_real : xbsIndex_r4/Slice  nbits=t+b  boolean_output=off  mode=Upper Bit Location + Width  bit1=0  base1=MSB of Input  bit0=0  base0=LSB of Input  dbl_ovrd=off  block_type=slice
  xWr : Outport
  xWi : Outport  Port=2
  wires:
  x_real/1 -> Reinterpret/1
  x_imaginary/1 -> Reinterpret1/1
  W_real/1 -> Mult1/2, Mult2/2
  x/1 -> x_real/1, x_imaginary/1
  Reinterpret/1 -> Mult/1, Mult2/1
  Reinterpret1/1 -> Mult1/1, Mult3/1
  W_imaginary/1 -> Mult/2, Mult3/2
  AddSub/1 -> xWi/1
  AddSub1/1 -> xWr/1
  Mult/1 -> AddSub/1
  Mult1/1 -> AddSub/2
  Mult3/1 -> AddSub1/2
  Mult2/1 -> AddSub1/1

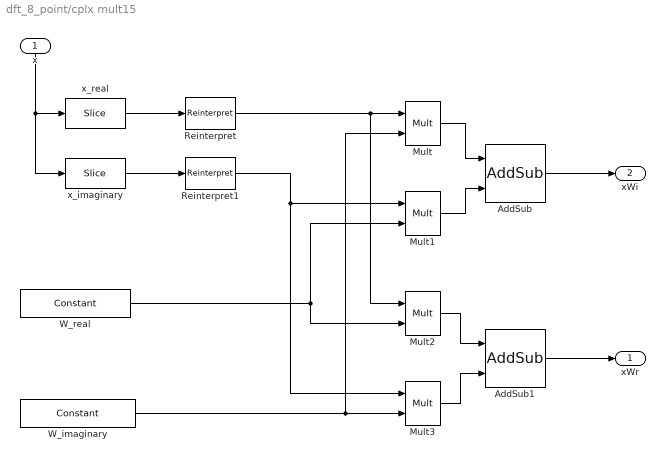
== system dft_8_point/cplx mult15 ==
  x : Inport
  AddSub : xbsIndex_r4/AddSub  mode=Addition  use_carryin=off  use_carryout=off  en=off  latency=0  precision=User Defined  arith_type="Signed  (2's comp)"  n_bits=t+b+1  bin_pt=b  quantization=Truncate  overflow=Wrap  use_behavioral_HDL=off  hw_selection=Fabric  pipelined=off  dbl_ovrd=off  block_type=addsub
  AddSub1 : xbsIndex_r4/AddSub  mode=Subtraction  use_carryin=off  use_carryout=off  en=off  latency=0  precision=User Defined  arith_type="Signed  (2's comp)"  n_bits=t+b+1  bin_pt=b  quantization=Truncate  overflow=Wrap  use_behavioral_HDL=off  hw_selection=Fabric  pipelined=off  dbl_ovrd=off  block_type=addsub
  Mult{,1..3} (4 alike) : xbsIndex_r4/Mult  precision=User Defined  arith_type="Signed  (2's comp)"  n_bits=t+b  bin_pt=b  quantization=Truncate  overflow=Wrap  en=off  latency=0  use_behavioral_HDL=off  opt=Speed  use_embedded=on  optimum_pipeline=off  pipeline=on  dbl_ovrd=off  use_rpm=on  placement_style=Triangular  block_type=mult
  Reinterpret : xbsIndex_r4/Reinterpret  force_arith_type=on  arith_type="Signed  (2's comp)"  force_bin_pt=on  bin_pt=b  block_type=reinterpret
      settings: infoedit="Changes signal type without altering the binary representation.   You can changed the signal between signed and unsigned, and relocate the binary point.<br><br>Hardware notes: In hardware this block costs nothing.<br><br>Example:  Suppose the input is 6 bits wide, signed, with 2 fractional bits, and the output is forced to unsigned with 0 fractional bits.  Then an input of -2.0 (1110.00 in binary 2's complement) becomes an output of 56 (111000 in binary)."
  Reinterpret1 : xbsIndex_r4/Reinterpret  force_arith_type=on  arith_type="Signed  (2's comp)"  force_bin_pt=on  bin_pt=b  block_type=reinterpret
      settings: infoedit="Changes signal type without altering the binary representation.   You can changed the signal between signed and unsigned, and relocate the binary point.<br><br>Hardware notes: In hardware this block costs nothing.<br><br>Example:  Suppose the input is 6 bits wide, signed, with 2 fractional bits, and the output is forced to unsigned with 0 fractional bits.  Then an input of -2.0 (1110.00 in binary 2's complement) becomes an output of 56 (111000 in binary)."
  W_imaginary : xbsIndex_r4/Constant  const=imag(Wnk)  gui_display_data_type=Fixed-point  arith_type=Signed (2's comp)  n_bits=t+b  bin_pt=b  preci_type=Single  exp_width=8  frac_width=24  explicit_period=off  period=1  equ=P=C  opselect=C  inp2=PCIN>>17  opr=+  inp1=P  carry=CIN  dbl_ovrd=off  block_type=constant
  W_real : xbsIndex_r4/Constant  const=real(Wnk)  gui_display_data_type=Fixed-point  arith_type=Signed (2's comp)  n_bits=t+b  bin_pt=b  preci_type=Single  exp_width=8  frac_width=24  explicit_period=off  period=1  equ=P=C  opselect=C  inp2=PCIN>>17  opr=+  inp1=P  carry=CIN  dbl_ovrd=off  block_type=constant
  x_imaginary : xbsIndex_r4/Slice  nbits=t+b  boolean_output=off  mode=Lower Bit Location + Width  bit1=0  base1=MSB of Input  bit0=0  base0=LSB of Input  dbl_ovrd=off  block_type=slice
  x_real : xbsIndex_r4/Slice  nbits=t+b  boolean_output=off  mode=Upper Bit Location + Width  bit1=0  base1=MSB of Input  bit0=0  base0=LSB of Input  dbl_ovrd=off  block_type=slice
  xWr : Outport
  xWi : Outport  Port=2
  wires:
  x_real/1 -> Reinterpret/1
  x_imaginary/1 -> Reinterpret1/1
  W_real/1 -> Mult1/2, Mult2/2
  x/1 -> x_real/1, x_imaginary/1
  Reinterpret/1 -> Mult/1, Mult2/1
  Reinterpret1/1 -> Mult1/1, Mult3/1
  W_imaginary/1 -> Mult/2, Mult3/2
  AddSub/1 -> xWi/1
  AddSub1/1 -> xWr/1
  Mult/1 -> AddSub/1
  Mult1/1 -> AddSub/2
  Mult3/1 -> AddSub1/2
  Mult2/1 -> AddSub1/1

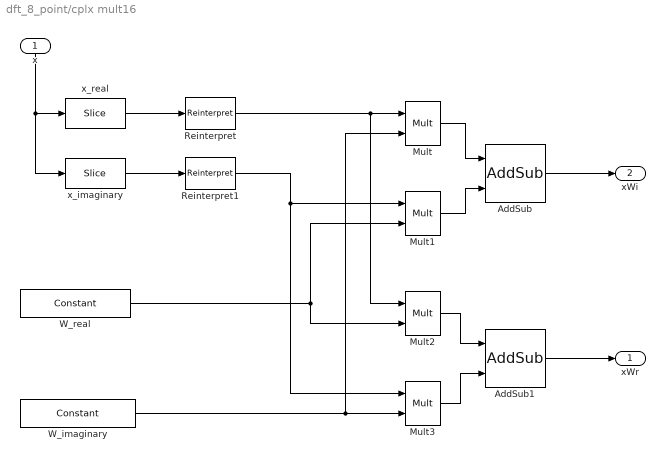
== system dft_8_point/cplx mult16 ==
  x : Inport
  AddSub : xbsIndex_r4/AddSub  mode=Addition  use_carryin=off  use_carryout=off  en=off  latency=0  precision=User Defined  arith_type="Signed  (2's comp)"  n_bits=t+b+1  bin_pt=b  quantization=Truncate  overflow=Wrap  use_behavioral_HDL=off  hw_selection=Fabric  pipelined=off  dbl_ovrd=off  block_type=addsub
  AddSub1 : xbsIndex_r4/AddSub  mode=Subtraction  use_carryin=off  use_carryout=off  en=off  latency=0  precision=User Defined  arith_type="Signed  (2's comp)"  n_bits=t+b+1  bin_pt=b  quantization=Truncate  overflow=Wrap  use_behavioral_HDL=off  hw_selection=Fabric  pipelined=off  dbl_ovrd=off  block_type=addsub
  Mult{,1..3} (4 alike) : xbsIndex_r4/Mult  precision=User Defined  arith_type="Signed  (2's comp)"  n_bits=t+b  bin_pt=b  quantization=Truncate  overflow=Wrap  en=off  latency=0  use_behavioral_HDL=off  opt=Speed  use_embedded=on  optimum_pipeline=off  pipeline=on  dbl_ovrd=off  use_rpm=on  placement_style=Triangular  block_type=mult
  Reinterpret : xbsIndex_r4/Reinterpret  force_arith_type=on  arith_type="Signed  (2's comp)"  force_bin_pt=on  bin_pt=b  block_type=reinterpret
      settings: infoedit="Changes signal type without altering the binary representation.   You can changed the signal between signed and unsigned, and relocate the binary point.<br><br>Hardware notes: In hardware this block costs nothing.<br><br>Example:  Suppose the input is 6 bits wide, signed, with 2 fractional bits, and the output is forced to unsigned with 0 fractional bits.  Then an input of -2.0 (1110.00 in binary 2's complement) becomes an output of 56 (111000 in binary)."
  Reinterpret1 : xbsIndex_r4/Reinterpret  force_arith_type=on  arith_type="Signed  (2's comp)"  force_bin_pt=on  bin_pt=b  block_type=reinterpret
      settings: infoedit="Changes signal type without altering the binary representation.   You can changed the signal between signed and unsigned, and relocate the binary point.<br><br>Hardware notes: In hardware this block costs nothing.<br><br>Example:  Suppose the input is 6 bits wide, signed, with 2 fractional bits, and the output is forced to unsigned with 0 fractional bits.  Then an input of -2.0 (1110.00 in binary 2's complement) becomes an output of 56 (111000 in binary)."
  W_imaginary : xbsIndex_r4/Constant  const=imag(Wnk)  gui_display_data_type=Fixed-point  arith_type=Signed (2's comp)  n_bits=t+b  bin_pt=b  preci_type=Single  exp_width=8  frac_width=24  explicit_period=off  period=1  equ=P=C  opselect=C  inp2=PCIN>>17  opr=+  inp1=P  carry=CIN  dbl_ovrd=off  block_type=constant
  W_real : xbsIndex_r4/Constant  const=real(Wnk)  gui_display_data_type=Fixed-point  arith_type=Signed (2's comp)  n_bits=t+b  bin_pt=b  preci_type=Single  exp_width=8  frac_width=24  explicit_period=off  period=1  equ=P=C  opselect=C  inp2=PCIN>>17  opr=+  inp1=P  carry=CIN  dbl_ovrd=off  block_type=constant
  x_imaginary : xbsIndex_r4/Slice  nbits=t+b  boolean_output=off  mode=Lower Bit Location + Width  bit1=0  base1=MSB of Input  bit0=0  base0=LSB of Input  dbl_ovrd=off  block_type=slice
  x_real : xbsIndex_r4/Slice  nbits=t+b  boolean_output=off  mode=Upper Bit Location + Width  bit1=0  base1=MSB of Input  bit0=0  base0=LSB of Input  dbl_ovrd=off  block_type=slice
  xWr : Outport
  xWi : Outport  Port=2
  wires:
  x_real/1 -> Reinterpret/1
  x_imaginary/1 -> Reinterpret1/1
  W_real/1 -> Mult1/2, Mult2/2
  x/1 -> x_real/1, x_imaginary/1
  Reinterpret/1 -> Mult/1, Mult2/1
  Reinterpret1/1 -> Mult1/1, Mult3/1
  W_imaginary/1 -> Mult/2, Mult3/2
  AddSub/1 -> xWi/1
  AddSub1/1 -> xWr/1
  Mult/1 -> AddSub/1
  Mult1/1 -> AddSub/2
  Mult3/1 -> AddSub1/2
  Mult2/1 -> AddSub1/1
